simulink model "ASK2"  (R2017a)
settings: Solver=VariableStepAuto  StartTime=0.0  RelTol=1e-3
libraries: dsparch4 x2, simulink x1, commrandsrc3 x1
settings Model: Creator=81228  LastModifiedBy=81228

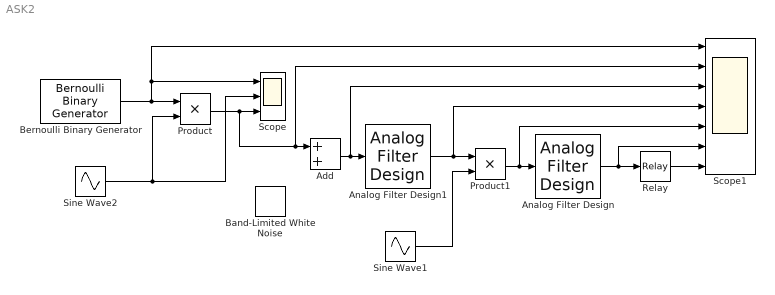
== system ASK2 ==
  Add : Sum
  Analog Filter Design : dsparch4/Analog Filter Design  method=Butterworth  filttype=Lowpass  N=2  Wlo=20*pi  Whi=80  Rp=2  Rs=40
  Analog Filter Design1 : dsparch4/Analog Filter Design  method=Butterworth  filttype=Bandpass  N=1  Wlo=180*pi  Whi=220*pi  Rp=2  Rs=40
  Band-Limited White Noise : simulink/Sources/Band-Limited White Noise  Cov=0.001  Ts=0.1  seed=[23341]
  Bernoulli Binary Generator : commrandsrc3/Bernoulli Binary Generator  ProbabilityOfZero=0.4  SeedSource=Parameter  Seed=61  SampleTime=0.1  SamplesPerFrame=1  OutputDataType=double  SimulateUsing=Interpreted execution
  Product : Product
  Product1 : Product
  Relay : Relay  OnSwitchValue=0.25  OffSwitchValue=0.25
  Scope : Scope  NumInputPorts=3
  Scope1 : Scope  NumInputPorts=7
  Sine Wave1 : Sin  Frequency=200*pi  SampleTime=1/10000
  Sine Wave2 : Sin  Frequency=200*pi  SampleTime=1/10000
  wires:
  Bernoulli Binary Generator/1 -> Scope/1, Scope1/1, Product/1
  Product/1 -> Scope1/2, Add/1, Scope/3
  Sine Wave2/1 -> Scope/2, Product/2
  Add/1 -> Scope1/3, Analog Filter Design1/1
  Analog Filter Design1/1 -> Scope1/4, Product1/1
  Product1/1 -> Scope1/5, Analog Filter Design/1
  Relay/1 -> Scope1/7
  Analog Filter Design/1 -> Relay/1, Scope1/6
  Sine Wave1/1 -> Product1/2
